simulink model "linea_recta_3D_SIM"  (R2020a)
settings: Solver=VariableStepAuto  StartTime=0.0  StopTime=45  RelTol=1e-3
InitFcn:
  | load('linea_recta_dataset.mat');
libraries: sim3dautolib x4, sim3dcameralib x1, sim3dlib x1
settings Model: EnablePacing=on  PacingRate=0.100000  Creator=derpb  LastModifiedBy=derpb

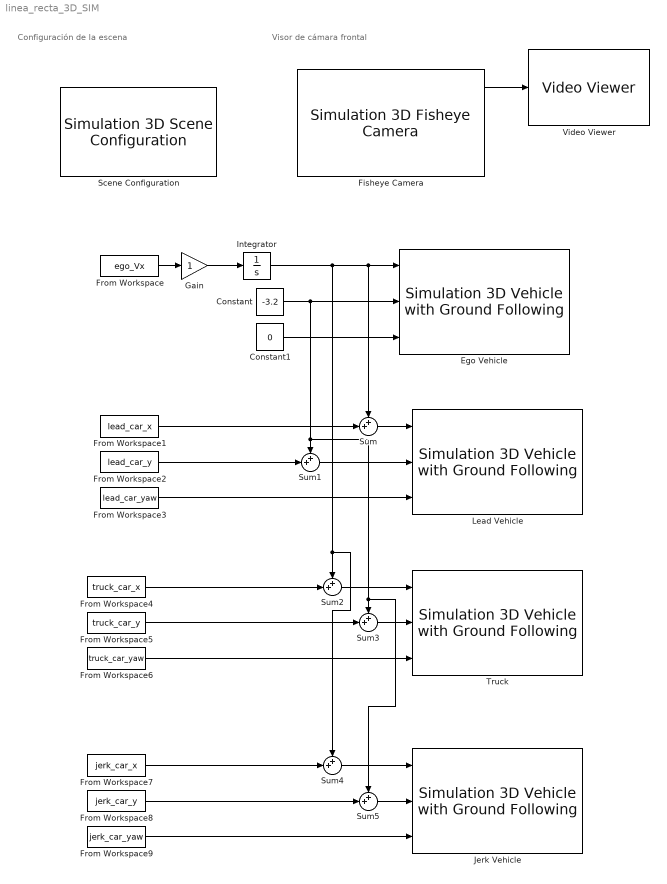
== system linea_recta_3D_SIM ==
  note: Visor de cámara frontal
  note: Configuración de la escena
  Constant : Constant  Value=-3.2
  Constant1 : Constant  Value=0
  Ego Vehicle : sim3dautolib/Simulation 3D Vehicle with Ground Following  Priority=-1  PassVehMesh=Muscle car  VehColor=Blue  InitialPos=[0, -3.2, 0]  InitialRot=[0, 0, 0]  ActorName=EgoCar  SampleTime=-1  ActorType=SimulinkVehicle  ID=C  aMode=3  ActorTag=EgoCar  CoordinateScheme=ISO  TransformOutportEnabled=off
      settings: SourceProductBaseCode=DR,VE
  Fisheye Camera : sim3dcameralib/Simulation 3D Fisheye Camera  Priority=1  sensorTag=Sim3dSensor1  sensorId=1  sensorName=Sim3dSensor1  vehTagList={'EgoCar';'Scene Origin'}  vehTag=EgoCar  mountLoc=Roof center  offsetFlag=off  tmountOffset=[0, 0, 0]  rmountOffset=[0, 0, 0]  OpticalCenter=[640, 360]  ImageSize=[720, 1280]  RadialDistortion=[320, 0, 0, 0]  TransformOutportEnabled=on  SampleTime=-1  mountPoint=[-0.25 0 1.57000005245209]  mountOrientation=[0 0 0]  aMode=3  ID=1
      settings: SourceProductBaseCode=DR,VE
  From Workspace : FromWorkspace  VariableName=ego_Vx  SampleTime=0.1
  From Workspace1 : FromWorkspace  VariableName=lead_car_x  SampleTime=-1
  From Workspace2 : FromWorkspace  VariableName=lead_car_y  SampleTime=-1
  From Workspace3 : FromWorkspace  VariableName=lead_car_yaw  SampleTime=-1
  From Workspace4 : FromWorkspace  VariableName=truck_car_x  SampleTime=-1
  From Workspace5 : FromWorkspace  VariableName=truck_car_y  SampleTime=-1
  From Workspace6 : FromWorkspace  VariableName=truck_car_yaw  SampleTime=-1
  From Workspace7 : FromWorkspace  VariableName=jerk_car_x  SampleTime=-1
  From Workspace8 : FromWorkspace  VariableName=jerk_car_y  SampleTime=-1
  From Workspace9 : FromWorkspace  VariableName=jerk_car_yaw  SampleTime=-1
  Gain : Gain
  Integrator : Integrator
  Jerk Vehicle : sim3dautolib/Simulation 3D Vehicle with Ground Following  Priority=-1  PassVehMesh=Hatchback  VehColor=Red  InitialPos=[-180, 0, 0]  InitialRot=[0, 0, 0]  ActorName=Jerk  SampleTime=-1  ActorType=SimulinkVehicle  ID=C  aMode=3  ActorTag=Jerk  CoordinateScheme=ISO  TransformOutportEnabled=off
      settings: SourceProductBaseCode=DR,VE
  Lead Vehicle : sim3dautolib/Simulation 3D Vehicle with Ground Following  Priority=-1  PassVehMesh=Sedan  VehColor=Orange  InitialPos=[80, -3.2, 0]  InitialRot=[0, 0, 0]  ActorName=Lead_vehicle  SampleTime=-1  ActorType=SimulinkVehicle  ID=C  aMode=3  ActorTag=Lead_vehicle  CoordinateScheme=ISO  TransformOutportEnabled=off
      settings: SourceProductBaseCode=DR,VE
  Scene Configuration : sim3dlib/Simulation 3D Scene Configuration  Priority=0  ProjectFormat=Default Scenes  SceneDesc=Straight road  ProjectName=VehicleSimulation.exe  ScenePath=/Game/Maps/HwStrght  vehTagList={'EgoCar';'Lead_vehicle';'Scene Origin'}  vehTag=EgoCar  OpVisEn=off  Ts=1/60  EnableWindow=on  sensorTag=MainCamera1  sensorId=1  sensorName=MainCamera1  mountLoc=Origin  offsetFlag=off  tmountOffset=[0, 0, 0]  rmountOffset=[0, 0, 0]  HorizontalResolution=1280  VerticalResolution=720  HorizontalFOV=60  mountPoint=[0 0 0]  mountOrientation=[0 0 0]  aMode=3  ID=1
      settings: SourceProductBaseCode=DR,VE
  Sum{,1..5} (6 alike) : Sum  Inputs=++|
  Truck : sim3dautolib/Simulation 3D Vehicle with Ground Following  Priority=-1  PassVehMesh=Box truck  VehColor=Green  InitialPos=[750, 0, 0]  InitialRot=[0, 0, 180]  ActorName=Truck  SampleTime=-1  ActorType=SimulinkVehicle  ID=C  aMode=3  ActorTag=Truck  CoordinateScheme=ISO  TransformOutportEnabled=off
      settings: SourceProductBaseCode=DR,VE
  Video Viewer : VideoViewer  FigPos=[1194 1032 569 528]
  wires:
  Fisheye Camera/1 -> Video Viewer/1
  From Workspace/1 -> Gain/1
  Constant/1 -> Sum5/1, Sum3/1, Sum1/1, Ego Vehicle/2
  Constant1/1 -> Ego Vehicle/3
  Gain/1 -> Integrator/1
  Integrator/1 -> Sum4/1, Sum2/1, Sum/1, Ego Vehicle/1
  Sum/1 -> Lead Vehicle/1
  Sum1/1 -> Lead Vehicle/2
  From Workspace2/1 -> Sum1/2
  From Workspace1/1 -> Sum/2
  From Workspace3/1 -> Lead Vehicle/3
  From Workspace6/1 -> Truck/3
  Sum2/1 -> Truck/1
  From Workspace4/1 -> Sum2/2
  From Workspace5/1 -> Sum3/2
  Sum3/1 -> Truck/2
  From Workspace7/1 -> Sum4/2
  Sum4/1 -> Jerk Vehicle/1
  Sum5/1 -> Jerk Vehicle/2
  From Workspace8/1 -> Sum5/2
  From Workspace9/1 -> Jerk Vehicle/3
